simulink model "Simulacao"  (R2013b)
settings: Solver=ode45  StartTime=0.0  StopTime=100  RelTol=1e-3
values from neighbouring files (symbols this model uses):
  A = [0    -2     0     0 ... (first row only)    [SYS.m]
  B = [1    0     0     0]'    [SYS.m]
  K = (rho^-1)*B'*F    [Target_System_ZP_LTR.m]
  Kdc = -1/(C*((A-B*K)^-1)*B)    [Target_System_ZP_LTR.m]
undefined symbols (not defined in the file or in its folder): C
settings Model: Creator=Eduardo  LastModifiedBy=Eduardo

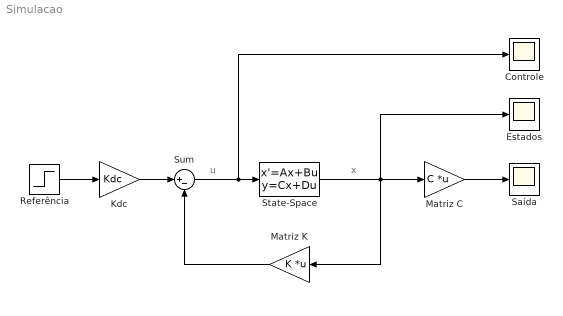
== system Simulacao ==
  note: u
  note: x
  Controle : Scope
      settings: SaveName=ScopeData2
  Estados : Scope
  Kdc : Gain  Gain=Kdc
  Matriz C : Gain  Gain=C  Multiplication=Matrix(K*u)
  Matriz K : Gain  Gain=K  Multiplication=Matrix(K*u)
  Referência : Step  SampleTime=0
  Saída : Scope
  State-Space : StateSpace  A=A  B=B  C=[eye(4)]  D=zeros(4,1)  X0=zeros(4,1)
  Sum : Sum  Inputs=|+-
  wires:
  State-Space/1 -> Matriz C/1, Matriz K/1, Estados/1
  Matriz C/1 -> Saída/1
  Sum/1 -> Controle/1, State-Space/1
  Matriz K/1 -> Sum/2
  Referência/1 -> Kdc/1
  Kdc/1 -> Sum/1
